simulink model "six_pulse_thyristor_rectifier"  (R2023b)
settings: Solver=VariableStepAuto  StartTime=0.0  StopTime=0.1  RelTol=1e-3
values from neighbouring files (symbols this model uses):
  a = 0    [init.m]
  T_s = 1/(2*f_s)    (= 6.25e-05)    [init.m]
  u_s = sqrt(2/3) * 150    [init.m]
  w0_pll = 2*pi*20    (= 125.663706144)    [init.m]
  w_n = 2*pi*50    (= 314.159265359)    [init.m]
undefined symbols (not defined in the file or in its folder): D1, lagging, plecs, pulse
libraries: slpidlib x1, spsPulseGeneratorThyristor6PulseLib x1, simulink x1
settings Model: Creator=chowd  LastModifiedBy=chowd

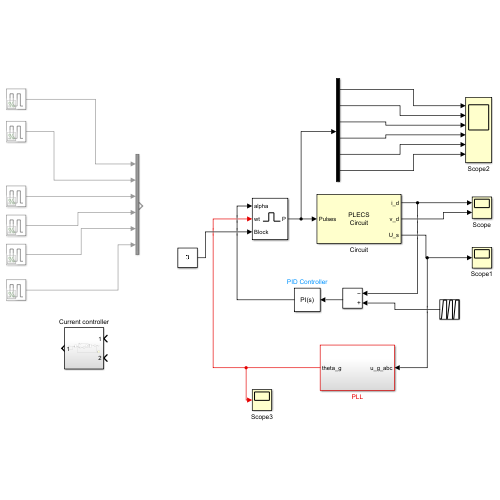
[thumbnail: Simulink's stored preview of the top-level diagram]
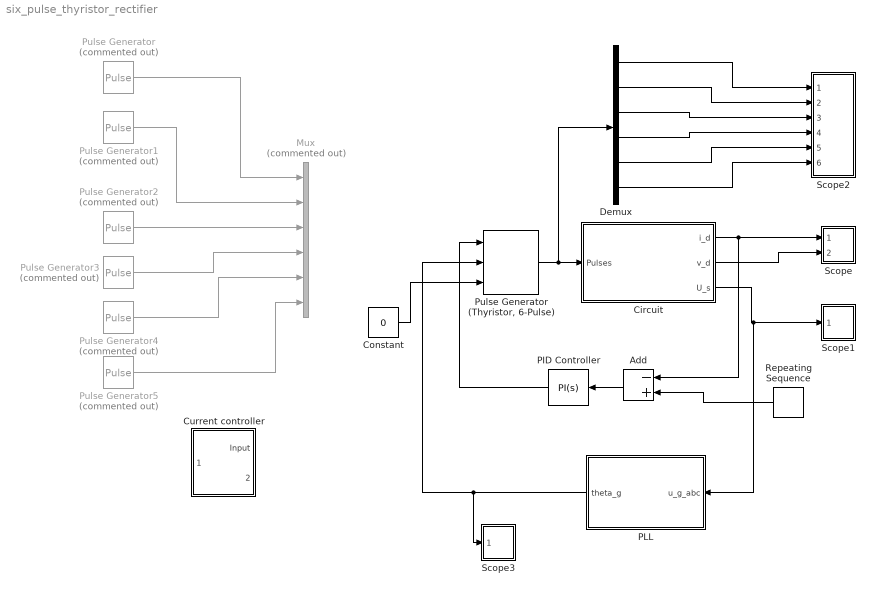
== system six_pulse_thyristor_rectifier ==
  Add : Sum  Inputs=-+
  Circuit : Subsystem  LoadFcn=plecs('sl', 200);  InitFcn=plecs('sl', 214);  StartFcn=plecs('sl', 208);  StopFcn=plecs('sl', 209);  mask(PlecsCircuit){PLECSData=<binary blob, 3244 chars, not shown>}
      mask prompts: PLECSData "PLECS Data (Do not delete or modify!)"
      mask init:
      | % PLACE CUSTOM INITIALIZATIONS ABOVE
      | % DO NOT REMOVE
      | plecs('sl', 215);
      | % DO NOT REMOVE
      settings: CopyFcn=plecs('sl', 203);  DeleteFcn=plecs('sl', 205);  UndoDeleteFcn=plecs('sl', 206);  PreSaveFcn=plecs('sl', 211);  PostSaveFcn=plecs('sl', 201);  NameChangeFcn=plecs('sl', 210);  DestroyFcn=plecs('sl', 207);  PreCopyFcn=plecs('sl', 216);  OpenFcn=plecs('sl', 202);  ErrorFcn=plerrorfcn
      mask Help: eval('plecs(''help'', ''qthelp:///creatingacircuit.html'')')
      mask Display: disp('PLECS\nCircuit')
  Constant : Constant  Value=0  SampleTime=T_s
  Current controller : Subsystem
  Demux : Demux  Outputs=6
  Mux : Mux  Commented=on  Inputs=6
  PID Controller : slpidlib/PID Controller  Controller=PI  Form=Parallel  TimeDomain=Continuous-time  UseExternalTs=off  SampleTime=-1  IntegratorMethod=Forward Euler  FilterMethod=Forward Euler  ControllerParametersSource=internal  P=10  I=5000  UseKiTs=off  D=0  N=100  UseFilter=on  TunerSelectOption=Transfer Function Based (PID Tuner App)  InitialConditionSource=internal  InitialConditionForIntegrator=0  InitialConditionForFilter=0  DifferentiatorICPrevScaledInput=0  ExternalReset=none  TrackingMode=off  Kt=1  LimitOutput=off  SatLimitsSource=internal  UpperSaturationLimit=160*pi/180  LowerSaturationLimit=pi/18  LinearizeAsGain=on  AntiWindupMode=none  Kb=1  LimitIntegrator=off  UpperIntegratorSaturationLimit=inf  LowerIntegratorSaturationLimit=-inf  POutMin=[]  POutMax=[]  IOutMin=[]  IOutMax=[]  DOutMin=[]  DOutMax=[]  NOutMin=[]  NOutMax=[]  SumOutMin=[]  SumOutMax=[]  SaturationOutMin=[]  SaturationOutMax=[]  PParamMin=[]  PParamMax=[]  IParamMin=[]  IParamMax=[]  DParamMin=[]  DParamMax=[]  NParamMin=[]  NParamMax=[]  KbParamMin=[]  KbParamMax=[]  KtParamMin=[]  KtParamMax=[]  KbOutMin=[]  KbOutMax=[]  KtOutMin=[]  KtOutMax=[]  IntegratorOutMin=[]  IntegratorOutMax=[]  FilterOutMin=[]  FilterOutMax=[]  SumI1OutMin=[]  SumI1OutMax=[]  SumI2OutMin=[]  SumI2OutMax=[]  SumI3OutMin=[]  SumI3OutMax=[]  SumI4OutMin=[]  SumI4OutMax=[]  SumDOutMin=[]  SumDOutMax=[]  DifferentiatorOutMin=[]  DifferentiatorOutMax=[]  FilterDiffOutCoefMin=[]  FilterDiffOutCoefMax=[]  ReciprocalOutMin=[]  ReciprocalOutMax=[]  SumDenOutMin=[]  SumDenOutMax=[]  SumNumOutMin=[]  SumNumOutMax=[]  DivideOutMin=[]  DivideOutMax=[]  UdiffTsProdOutMin=[]  UdiffTsProdOutMax=[]  NTsProdOutMin=[]  NTsProdOutMax=[]  UintegralTsProdOutMin=[]  UintegralTsProdOutMax=[]  UngainTsProdOutMin=[]  UngainTsProdOutMax=[]  ClampingZeroOutDataTypeStr=Inherit: Inherit via back propagation  ClampingZeroOutMin=[]  ClampingZeroOutMax=[]  FilterDenConstantOutDataTypeStr=Inherit: Inherit via back propagation  FilterDenConstantOutMin=[]  FilterDenConstantOutMax=[]  PCopyOutDataTypeStr=Inherit: Inherit via back propagation  PCopyOutMin=[]  PCopyOutMax=[]  NCopyOutDataTypeStr=Inherit: Inherit via back propagation  NCopyOutMin=[]  NCopyOutMax=[]  IntegratorContinuousStateAttributes=''  IntegratorStateMustResolveToSignalObject=off  IntegratorRTWStateStorageClass=Auto  FilterContinuousStateAttributes=''  FilterStateMustResolveToSignalObject=off  FilterRTWStateStorageClass=Auto  ParallelPVariant=InternalParameters  IdealPVariant=Disabled  IVariant=InternalParameters  DVariant=Disabled  IntegratorVariant=Continuous  SatVariant=Disabled  AWVariant=Passthrough  PCopyVariant=Disabled  TRVariant=Disabled  FdbkBlocksVariant=Forward  IdealPFdbkVariant=Disabled  SatFdbkVariant=Disabled  DerivativeFilterVariant=Disabled  NVariant=Disabled  NCopyVariant=Disabled_SignalSpec  FilterICVariant=Disabled  IntegratorICVariant=InternalICs  ExternalResetVariant=Disabled  TRSumVariant=Passthrough  SumFdbkVariant=Disabled  SumVariant=Sum_PI  TsampFilterVariant=InternalTs  TsampNgainVariant=Passthrough  TsampIntegralVariant=Disabled_SignalSpec  ExternalSaturationOutDataTypeStr=Inherit: Same as second input
  PLL : Subsystem
  Pulse Generator : DiscretePulseGenerator  Commented=on  PulseType=Time based  Period=T_s  PulseWidth=16.67  PhaseDelay=a*T_s/360
  Pulse Generator1 : DiscretePulseGenerator  Commented=on  PulseType=Time based  Period=T_s  PulseWidth=16.67  PhaseDelay=(a+60)*T_s/360
  Pulse Generator2 : DiscretePulseGenerator  Commented=on  PulseType=Time based  Period=T_s  PulseWidth=16.67  PhaseDelay=(a+120)*T_s/360
  Pulse Generator3 : DiscretePulseGenerator  Commented=on  PulseType=Time based  Period=T_s  PulseWidth=16.67  PhaseDelay=(a+180)*T_s/360
  Pulse Generator4 : DiscretePulseGenerator  Commented=on  PulseType=Time based  Period=T_s  PulseWidth=16.67  PhaseDelay=(a+240)*T_s/360
  Pulse Generator5 : DiscretePulseGenerator  Commented=on  PulseType=Time based  Period=T_s  PulseWidth=16.67  PhaseDelay=(a+300)*T_s/360
  "Pulse Generator (Thyristor, 6-Pulse)" : spsPulseGeneratorThyristor6PulseLib/Pulse Generator (Thyristor, 6-Pulse)  GenType=6-pulse  Delta=D1 (lagging)  pwidth=180  Double_Pulse=off  Ts=T_s
      settings: LibrarySourceBlock=|
      | sps_lib/Power Electronics/Power Electronics Control/Pulse Generator
      | (Thyristor, 6-Pulse)
  Repeating Sequence : simulink/Sources/Repeating Sequence  rep_seq_t=[0 10 30 60]*1e-3  rep_seq_y=[0 0 1 1]*1e3
  Scope : Subsystem  LoadFcn=plecs('sl', 300);  InitFcn=plecs('sl', 314);  StartFcn=plecs('sl', 308);  StopFcn=plecs('sl', 309);  mask{Settings=<binary blob, 1192 chars, not shown>}
      mask init:
      | plecs('sl', 315);
      settings: CopyFcn=plecs('sl', 303);  DeleteFcn=plecs('sl', 305);  UndoDeleteFcn=plecs('sl', 306);  PreSaveFcn=plecs('sl', 311);  NameChangeFcn=plecs('sl', 310);  DestroyFcn=plecs('sl', 307);  OpenFcn=plecs('sl', 302);  ErrorFcn=plerrorfcn
      mask Display: plot([0.1 0.9 0.9 0.1 0.1], [0.9 0.9 0.5 0.5 0.9])
  Scope1 : Subsystem  LoadFcn=plecs('sl', 300);  InitFcn=plecs('sl', 314);  StartFcn=plecs('sl', 308);  StopFcn=plecs('sl', 309);  mask{Settings=<binary blob, 1052 chars, not shown>}
      mask init:
      | plecs('sl', 315);
      settings: CopyFcn=plecs('sl', 303);  DeleteFcn=plecs('sl', 305);  UndoDeleteFcn=plecs('sl', 306);  PreSaveFcn=plecs('sl', 311);  NameChangeFcn=plecs('sl', 310);  DestroyFcn=plecs('sl', 307);  OpenFcn=plecs('sl', 302);  ErrorFcn=plerrorfcn
      mask Display: plot([0.1 0.9 0.9 0.1 0.1], [0.9 0.9 0.5 0.5 0.9])
  Scope2 : Subsystem  LoadFcn=plecs('sl', 300);  InitFcn=plecs('sl', 314);  StartFcn=plecs('sl', 308);  StopFcn=plecs('sl', 309);  mask{Settings=<binary blob, 1748 chars, not shown>}
      mask init:
      | plecs('sl', 315);
      settings: CopyFcn=plecs('sl', 303);  DeleteFcn=plecs('sl', 305);  UndoDeleteFcn=plecs('sl', 306);  PreSaveFcn=plecs('sl', 311);  NameChangeFcn=plecs('sl', 310);  DestroyFcn=plecs('sl', 307);  OpenFcn=plecs('sl', 302);  ErrorFcn=plerrorfcn
      mask Display: plot([0.1 0.9 0.9 0.1 0.1], [0.9 0.9 0.5 0.5 0.9])
  Scope3 : Subsystem  LoadFcn=plecs('sl', 300);  InitFcn=plecs('sl', 314);  StartFcn=plecs('sl', 308);  StopFcn=plecs('sl', 309);  mask{Settings=<binary blob, 1052 chars, not shown>}
      mask init:
      | plecs('sl', 315);
      settings: CopyFcn=plecs('sl', 303);  DeleteFcn=plecs('sl', 305);  UndoDeleteFcn=plecs('sl', 306);  PreSaveFcn=plecs('sl', 311);  NameChangeFcn=plecs('sl', 310);  DestroyFcn=plecs('sl', 307);  OpenFcn=plecs('sl', 302);  ErrorFcn=plerrorfcn
      mask Display: plot([0.1 0.9 0.9 0.1 0.1], [0.9 0.9 0.5 0.5 0.9])
  wires:
  Pulse Generator1/1 -> Mux/2
  Pulse Generator2/1 -> Mux/3
  Pulse Generator3/1 -> Mux/4
  Pulse Generator4/1 -> Mux/5
  Pulse Generator5/1 -> Mux/6
  Pulse Generator/1 -> Mux/1
  Circuit/1(i_d) -> Add/1, Scope/1(1)
  Circuit/2(v_d) -> Scope/2(2)
  Circuit/3(U_s) -> PLL/1(u_g_abc), Scope1/1(1)
  "Pulse Generator (Thyristor, 6-Pulse)"/1 -> Demux/1, Circuit/1(Pulses)
  PLL/1(theta_g) -> "Pulse Generator (Thyristor, 6-Pulse)"/2, Scope3/1(1)
  Constant/1 -> "Pulse Generator (Thyristor, 6-Pulse)"/3
  Demux/1 -> Scope2/1(1)
  Demux/2 -> Scope2/2(2)
  Demux/3 -> Scope2/3(3)
  Demux/4 -> Scope2/4(4)
  Demux/5 -> Scope2/5(5)
  Demux/6 -> Scope2/6(6)
  Add/1 -> PID Controller/1
  PID Controller/1 -> "Pulse Generator (Thyristor, 6-Pulse)"/1
  Repeating Sequence/1 -> Add/2

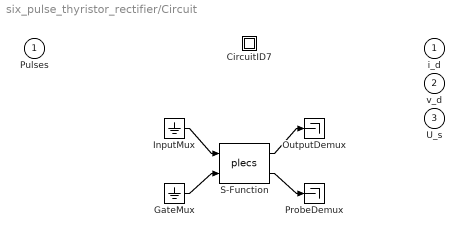
== system six_pulse_thyristor_rectifier/Circuit ==
  Pulses : Inport  PortDimensions=6
  " CircuitID7 " : Subsystem
  " GateMux " : Ground
  " InputMux " : Ground
  " OutputDemux " : Terminator
  " ProbeDemux " : Terminator
  " S-Function " : S-Function  FunctionName=plecs  SFunctionDeploymentMode=off  EnableBusSupport=off
  i_d : Outport  PortDimensions=1
  v_d : Outport  Port=2  PortDimensions=1
  U_s : Outport  Port=3  PortDimensions=3
  wires:
  " InputMux "/1 -> " S-Function "/1
  " GateMux "/1 -> " S-Function "/2
  " S-Function "/1 -> " OutputDemux "/1
  " S-Function "/2 -> " ProbeDemux "/1

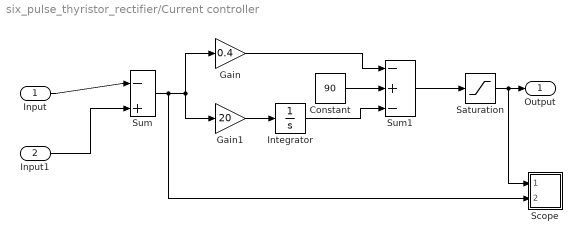
== system six_pulse_thyristor_rectifier/Current controller ==
  Input : Inport
  Input1 : Inport  Port=2
  Constant : Constant  Value=90  SampleTime=T_s
  Gain : Gain  Gain=0.4
  Gain1 : Gain  Gain=20
  Integrator : Integrator
  Saturation : Saturate  UpperLimit=162  LowerLimit=18
  Scope : Subsystem  LoadFcn=plecs('sl', 300);  InitFcn=plecs('sl', 314);  StartFcn=plecs('sl', 308);  StopFcn=plecs('sl', 309);  mask{Settings=<binary blob, 1192 chars, not shown>}
      mask init:
      | plecs('sl', 315);
      settings: CopyFcn=plecs('sl', 303);  DeleteFcn=plecs('sl', 305);  UndoDeleteFcn=plecs('sl', 306);  PreSaveFcn=plecs('sl', 311);  NameChangeFcn=plecs('sl', 310);  DestroyFcn=plecs('sl', 307);  OpenFcn=plecs('sl', 302);  ErrorFcn=plerrorfcn
      mask Display: plot([0.1 0.9 0.9 0.1 0.1], [0.9 0.9 0.5 0.5 0.9])
  Sum : Sum  Inputs=|-+
  Sum1 : Sum  Inputs=-+-
  Output : Outport
  wires:
  Sum/1 -> Scope/2(2), Gain1/1, Gain/1
  Constant/1 -> Sum1/2
  Gain/1 -> Sum1/1
  Gain1/1 -> Integrator/1
  Integrator/1 -> Sum1/3
  Sum1/1 -> Saturation/1
  Saturation/1 -> Scope/1(1), Output/1
  Input/1 -> Sum/1
  Input1/1 -> Sum/2

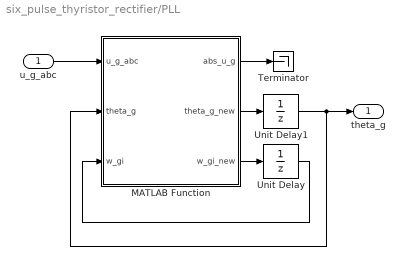
== system six_pulse_thyristor_rectifier/PLL ==
  u_g_abc : Inport
  MATLAB Function : MATLAB Function  TreatAsAtomicUnit=on
  Terminator : Terminator
  Unit Delay : UnitDelay  InitialCondition=w_n  SampleTime=-1  HasFrameUpgradeWarning=on
  Unit Delay1 : UnitDelay  SampleTime=-1  HasFrameUpgradeWarning=on
  theta_g : Outport
  wires:
  u_g_abc/1 -> MATLAB Function/1(u_g_abc)
  MATLAB Function/3(w_gi_new) -> Unit Delay/1
  MATLAB Function/2(theta_g_new) -> Unit Delay1/1
  Unit Delay1/1 -> MATLAB Function/2(theta_g), theta_g/1
  Unit Delay/1 -> MATLAB Function/3(w_gi)
  MATLAB Function/1(abs_u_g) -> Terminator/1

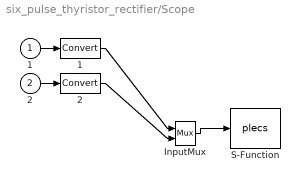
== system six_pulse_thyristor_rectifier/Scope ==
  1 : Inport
  2 : Inport  Port=2
  " 1 " : DataTypeConversion
  " 2 " : DataTypeConversion
  " InputMux " : Mux  Inputs=2
  " S-Function " : S-Function  FunctionName=plecs  SFunctionDeploymentMode=off  EnableBusSupport=off
  wires:
  " InputMux "/1 -> " S-Function "/1
  1/1 -> " 1 "/1
  " 1 "/1 -> " InputMux "/1
  2/1 -> " 2 "/1
  " 2 "/1 -> " InputMux "/2

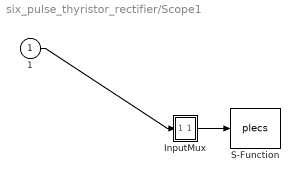
== system six_pulse_thyristor_rectifier/Scope1 ==
  1 : Inport
  " InputMux " : Subsystem
      mask Display: disp('Mux')
  " S-Function " : S-Function  FunctionName=plecs  SFunctionDeploymentMode=off  EnableBusSupport=off
  wires:
  1/1 -> " InputMux "/1(In1)
  " InputMux "/1(Out) -> " S-Function "/1

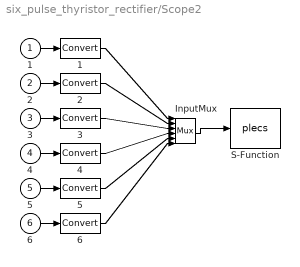
== system six_pulse_thyristor_rectifier/Scope2 ==
  1 : Inport
  2 : Inport  Port=2
  3 : Inport  Port=3
  4 : Inport  Port=4
  5 : Inport  Port=5
  6 : Inport  Port=6
  " 1 " : DataTypeConversion
  " 2 " : DataTypeConversion
  " 3 " : DataTypeConversion
  " 4 " : DataTypeConversion
  " 5 " : DataTypeConversion
  " 6 " : DataTypeConversion
  " InputMux " : Mux  Inputs=6
  " S-Function " : S-Function  FunctionName=plecs  SFunctionDeploymentMode=off  EnableBusSupport=off
  wires:
  " InputMux "/1 -> " S-Function "/1
  1/1 -> " 1 "/1
  " 1 "/1 -> " InputMux "/1
  2/1 -> " 2 "/1
  " 2 "/1 -> " InputMux "/2
  3/1 -> " 3 "/1
  " 3 "/1 -> " InputMux "/3
  4/1 -> " 4 "/1
  " 4 "/1 -> " InputMux "/4
  5/1 -> " 5 "/1
  " 5 "/1 -> " InputMux "/5
  6/1 -> " 6 "/1
  " 6 "/1 -> " InputMux "/6

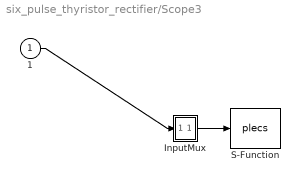
== system six_pulse_thyristor_rectifier/Scope3 ==
  1 : Inport
  " InputMux " : Subsystem
      mask Display: disp('Mux')
  " S-Function " : S-Function  FunctionName=plecs  SFunctionDeploymentMode=off  EnableBusSupport=off
  wires:
  1/1 -> " InputMux "/1(In1)
  " InputMux "/1(Out) -> " S-Function "/1

== system six_pulse_thyristor_rectifier/Circuit/ CircuitID7  ==

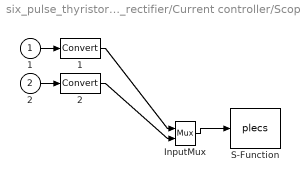
== system six_pulse_thyristor_rectifier/Current controller/Scope ==
  1 : Inport
  2 : Inport  Port=2
  " 1 " : DataTypeConversion
  " 2 " : DataTypeConversion
  " InputMux " : Mux  Inputs=2
  " S-Function " : S-Function  FunctionName=plecs  SFunctionDeploymentMode=off  EnableBusSupport=off
  wires:
  " InputMux "/1 -> " S-Function "/1
  1/1 -> " 1 "/1
  " 1 "/1 -> " InputMux "/1
  2/1 -> " 2 "/1
  " 2 "/1 -> " InputMux "/2

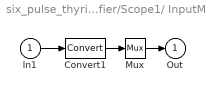
== system six_pulse_thyristor_rectifier/Scope1/ InputMux  ==
  In1 : Inport
  Convert1 : DataTypeConversion
  Mux : Mux  Inputs=1
  Out : Outport
  wires:
  Convert1/1 -> Mux/1
  In1/1 -> Convert1/1
  Mux/1 -> Out/1

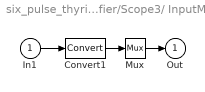
== system six_pulse_thyristor_rectifier/Scope3/ InputMux  ==
  In1 : Inport
  Convert1 : DataTypeConversion
  Mux : Mux  Inputs=1
  Out : Outport
  wires:
  Convert1/1 -> Mux/1
  In1/1 -> Convert1/1
  Mux/1 -> Out/1

== matlab function six_pulse_thyristor_rectifier/PLL/MATLAB Function ==
  settings: updateMethod=DISCRETE  sampleTime=T_s
  data: u_g_abc input size=3; theta_g input; w_gi input; u_s parameter; w0_pll parameter; abs_u_g output size=1; theta_g_new output; w_gi_new output; T_s parameter
function [abs_u_g, theta_g_new, w_gi_new] = pll(u_g_abc, ...
    theta_g, w_gi, u_s, w0_pll, T_s)

% Parameters 
% (Tuning of the PLL is analogous to that of the DC-voltage controller.)
zeta = 1;   % Damping ratio
k_p = 2*zeta*w0_pll/u_s; 
k_i = w0_pll^2/u_s;

% Space-vector transformation from phase-to-neutral components
u_gs = 2/3*(u_g_abc(1) + u_g_abc(2)*exp(1j*2*pi/3) + u_g_abc(3)*exp(1j*4*pi/3));

% Coordinate transformation to the "estimated" grid coordinates
u_g = exp(-1j*theta_g)*u_gs;

% Error signal, which is drive to zero by the PLL
u_gq = imag(u_g);

w_g = k_p*u_gq + w_gi;

% Update the integral state
w_gi_new = w_gi + T_s*k_i*u_gq;

% Update the grid-voltage angle
theta_g_new = theta_g + T_s*w_g;
while(theta_g_new > 2*pi)
     theta_g_new = theta_g_new - 2*pi;
end
while(theta_g_new < 0)
     theta_g_new = theta_g_new + 2*pi;
end

% Absolute value of the grid-voltage vector
abs_u_g = abs(u_g);
